simulink model "SimulacionTarea2"  (R2023b)
settings: Solver=ode8  StartTime=0.0  StopTime=1  RelTol=1e-3
settings Model: Creator=Lenovo  LastModifiedBy=Lenovo

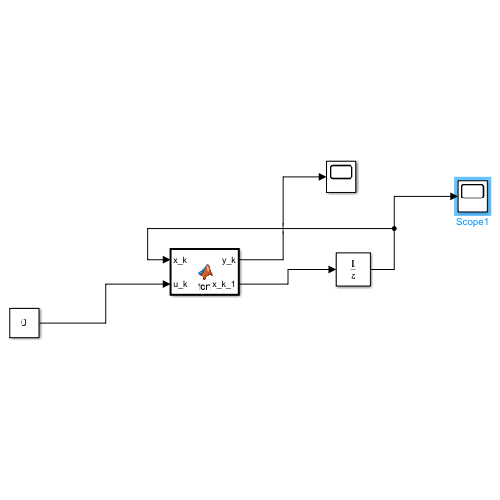
[thumbnail: Simulink's stored preview of the top-level diagram]
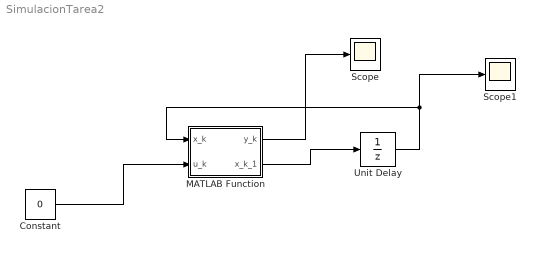
== system SimulacionTarea2 ==
  Constant : Constant  Value=0
  MATLAB Function : MATLAB Function  TreatAsAtomicUnit=on
  Scope : Scope
  Scope1 : Scope
  Unit Delay : UnitDelay  InitialCondition=[0.1; 0.1; 0.1]  SampleTime=-1  HasFrameUpgradeWarning=on
  wires:
  Constant/1 -> MATLAB Function/2(u_k)
  MATLAB Function/2(x_k_1) -> Unit Delay/1
  Unit Delay/1 -> Scope1/1, MATLAB Function/1(x_k)
  MATLAB Function/1(y_k) -> Scope/1

== matlab function SimulacionTarea2/MATLAB Function ==
  data: x_k input; y_k output; u_k input; x_k_1 output
function [y_k, x_k_1]=fcn(x_k, u_k)
A = (1/4)*[0 0 1; -4 1 4;0 0 -1];
B = [0;1;0];
C=[1 1 0];
x_k_1=A*x_k + B*u_k;
y_k= C*x_k;
